simulink model "A421_Final_Proj_detumble_deliv3"  (R2023a)
settings: Solver=VariableStepAuto  StartTime=0.0  StopTime=tspan  RelTol=1e-3
values from neighbouring files (symbols this model uses):
  k = k+1    (= 1)    [A421_FinalProj_MainScript.m]    (also in WheelSizing_Script.m)
undefined symbols (not defined in the file or in its folder): J, normal
settings Model: Creator=jself  LastModifiedBy=jself
settings DebuggingCC: UnconnectedInputMsg=warning  UnconnectedOutputMsg=warning  UnconnectedLineMsg=warning
settings ModelReferenceCC: EnableRefExpFcnMdlSchedulingChecks=on
settings RTWCC: DLArmComputeVersion=19.05

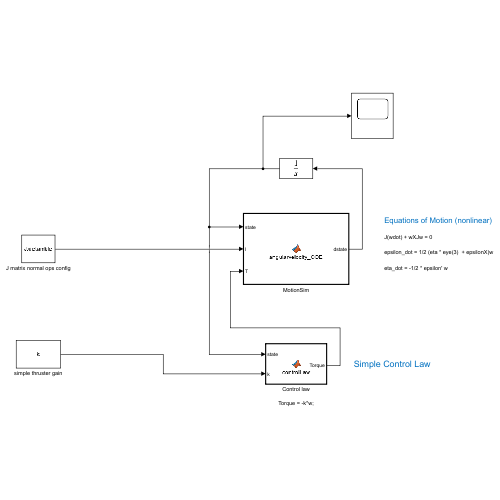
[thumbnail: Simulink's stored preview of the top-level diagram]
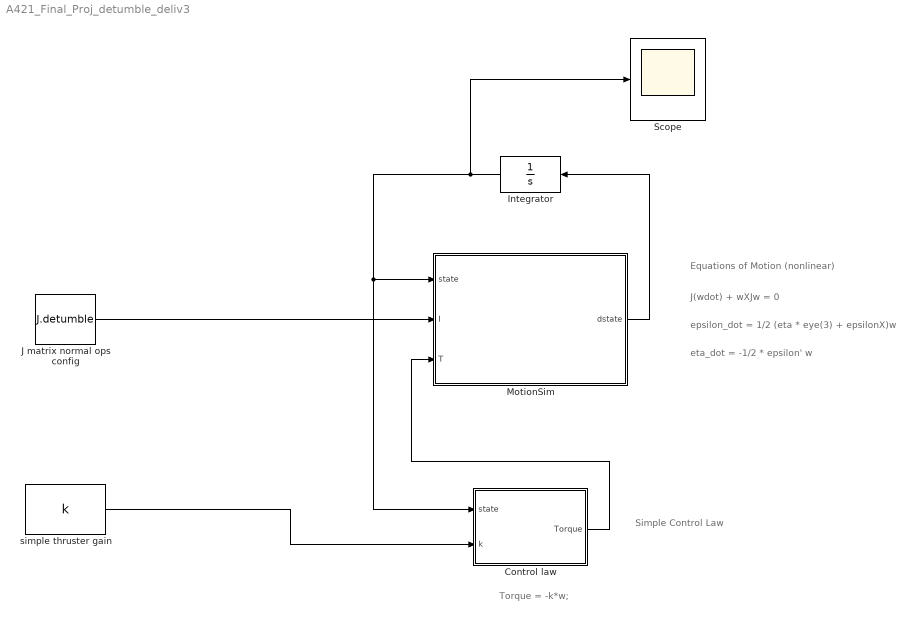
== system A421_Final_Proj_detumble_deliv3 ==
  note: Simple Control Law
  note: Torque = -k*w;
  note: Equations of Motion (nonlinear)
  note: eta_dot = -1/2 * epsilon' w
  note: epsilon_dot = 1/2 (eta * eye(3) + epsilonX)w
  note: J(wdot) + wXJw = 0
  Control law : MATLAB Function  TreatAsAtomicUnit=on
  Integrator : Integrator  InitialCondition=normal.state
  J matrix normal ops config : Constant  Value=J.detumble
  MotionSim : MATLAB Function  TreatAsAtomicUnit=on
  Scope : Scope
  simple thruster gain : Constant  Value=k
  wires:
  MotionSim/1(dstate) -> Integrator/1
  Integrator/1 -> Control law/1(state), MotionSim/1(state), Scope/1
  J matrix normal ops config/1 -> MotionSim/2(I)
  simple thruster gain/1 -> Control law/2(k)
  Control law/1(Torque) -> MotionSim/3(T)

== matlab function A421_Final_Proj_detumble_deliv3/MotionSim ==
  data: state input; dstate output; I input; T input
function dstate  = angularvelocity_ODE(state,I,T)

%{
This function is created for use in MATLAB's ode45 solver to compute the
following: 
    i.      Euler angle changes with time
    ii.     Quaternion changes with time
    iii.    Omega dot (change in angular velocity w.r.t time

INPUTS: 
    time = timespan for ode45
    state = mega state vector that contains all pertinent initial
    conditions. I.E., [omega; eulerangles, quaternion] 

state(1) = wx
state(2) = wy
state(3) = wz
state(4) = phi
state(5) = theta
state(6) = psi
state(7) = epsilonx
state(8) = epsilony
state(9) = epsilonz
state(10) = eta

I = inertia matrix (3x3) for the rigid body under consideration
T = net external torque (col vect) for system


OUTPUTS: derivative of the state for ode45 computation.
%}

%% Omega Dot
% The relationship for wdot needs:
    % i. center of mass inertia matrix I
    % ii. omega cross matrix

    w = [state(1);
         state(2);
         state(3)];

% Find omega cross matrix
w_cross =   [   0      -w(3)     w(2);
                w(3)    0        -w(1);
               -w(2)    w(1)      0   ];

wdot = inv(I) * (T - w_cross * I * w);

%dstate(1:3) = wdot;

%% Euler Angles

phi = state(4);
theta = state(5);
psi = state(6);

eulerdot = cos(theta)^(-1) * [   cos(theta)      sin(phi)*sin(theta)     cos(phi)*sin(theta); 
                                0               cos(phi)*cos(theta)     -sin(phi)*cos(theta);
                                0               sin(phi)                 cos(phi)           ] * w;

%% Quaternion Parameterization

epx = state(7);
epy = state(8);
epz = state(9);
eta = state(10);

epsilon = [epx; epy; epz];

epsilon_cross = [   0       -epz     epy;
                    epz     0        -epx;
                    -epy    epx      0    ];

% Derivatives of epsilon and eta
depsilon = 0.5 * (eta*eye(3) + epsilon_cross) * w;
deta = -0.5 * epsilon' * w;

% tell matlab to integrate this 
% MUST BE COLUMN VECT for ode45 to work

quat = [depsilon(1); depsilon(2); depsilon(3); deta];

dstate = [wdot;eulerdot;quat];

end

== matlab function A421_Final_Proj_detumble_deliv3/Control law ==
  data: state input; k input; Torque output
function Torque = controlLaw(state,k)

w = [state(1); state(2); state(3)];
Torque = -k*w;

end
